simulink model "ADCS_onOrbit_TrueState"  (R2024b)
settings: Solver=ode4  StartTime=0.0  StopTime=tspan  FixedStep=1  RelTol=1e-3
undefined symbols (not defined in the file): A_list, A_m, A_w, CD, COP, dYear, eta, J_body, J_wheels, JD0, K_d, K_p, K_w, m, mag_moment, mode, mu, n_list, p, period, q1_ini, q2_ini, q3_ini, q4_ini, r_I_ini, rE, sigma_B, sigma_b, sigma_g, sigma_S, v_I_ini, wB_1, wB_2, wB_3, wE, wW_1, wW_2, wW_3
libraries: simulink_extras x12, matrix_library x3, sharedtransform x3, simulink x1
(part 2 of 2)

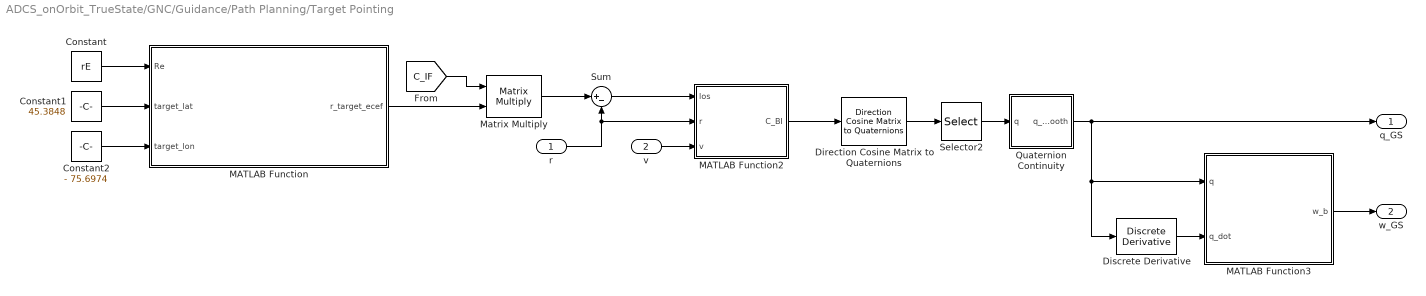
== system ADCS_onOrbit_TrueState/GNC/Guidance/Path Planning/Target Pointing ==
  r : Inport
  v : Inport  Port=2
  Constant : Constant  Value=rE
  Constant1 : Constant  Value=45.3848
  Constant2 : Constant  Value=- 75.6974
  Direction Cosine Matrix to Quaternions : sharedtransform/Direction Cosine Matrix  to Quaternions  aMode=0  action=None  tolerance=eps(2)
      settings: LibrarySourceBlock=|
      | aerolibtransform2/Direction Cosine Matrix
      | to Quaternions
  Discrete Derivative : simulink/Discrete/Discrete Derivative  gainval=1.0  ICPrevScaledInput=0.0  OutMin=[]  OutMax=[]  OutDataType=fixdt(1, 16)  OutScaling=2^-10  DoSatur=off
  MATLAB Function : MATLAB Function  TreatAsAtomicUnit=on
  MATLAB Function2 : MATLAB Function  TreatAsAtomicUnit=on
  MATLAB Function3 : MATLAB Function  TreatAsAtomicUnit=on
  Matrix Multiply : Product  Multiplication=Matrix(*)
  Quaternion Continuity : Subsystem
      mask Display: disp('Quaternion\nContinuity');
  Selector2 : Selector  InputPortWidth=4  IndexOptions=Index vector (dialog)  Indices=[2 3 4 1]  OutputSizes=1
  Sum : Sum  Inputs=|+-
  q_GS : Outport
  w_GS : Outport  Port=2
  wires:
  Constant/1 -> MATLAB Function/1(Re)
  Constant1/1 -> MATLAB Function/2(target_lat)
  Constant2/1 -> MATLAB Function/3(target_lon)
  MATLAB Function/1(r_target_ecef) -> Matrix Multiply/2
  Matrix Multiply/1 -> Sum/1
  r/1 -> MATLAB Function2/2(r), Sum/2
  Sum/1 -> MATLAB Function2/1(los)
  MATLAB Function2/1(C_BI) -> Direction Cosine Matrix to Quaternions/1
  Direction Cosine Matrix to Quaternions/1 -> Selector2/1
  Selector2/1 -> Quaternion Continuity/1(q)
  Quaternion Continuity/1(q_smooth) -> MATLAB Function3/1(q), Discrete Derivative/1, q_GS/1
  Discrete Derivative/1 -> MATLAB Function3/2(q_dot)
  MATLAB Function3/1(w_b) -> w_GS/1
  v/1 -> MATLAB Function2/3(v)
  [C_IF] -> Matrix Multiply/1

== system ADCS_onOrbit_TrueState/GNC/Navigation/TRIAD Determination/Quaternion Continuity ==
  q : Inport
  MATLAB Function2 : MATLAB Function  TreatAsAtomicUnit=on
  Unit Delay1 : UnitDelay  InitialCondition=[0 0 0 1]'  SampleTime=-1  HasFrameUpgradeWarning=on
  q_smooth : Outport
  wires:
  MATLAB Function2/1(q_smooth) -> q_smooth/1, Unit Delay1/1
  Unit Delay1/1 -> MATLAB Function2/2(q_prev)
  q/1 -> MATLAB Function2/1(q)

== system ADCS_onOrbit_TrueState/RWP/Environment/Variant Subsystem/ENV ==
  C_BI : Inport
  s : Inport  Port=2
  state : Inport  Port=3
  Drag : Subsystem
  Gravity Gradient : Subsystem
  Mag Torque : Subsystem
  Selector : Selector  InputPortWidth=6  IndexOptions=Index vector (dialog)  Indices=[1 2 3]  OutputSizes=1
  Selector1 : Selector  InputPortWidth=6  IndexOptions=Index vector (dialog)  Indices=[4 5 6]  OutputSizes=1
  Solar Radiation Pressure : Subsystem
  Sum : Sum  Inputs=++++
  B_b : Outport
  T_ext : Outport  Port=2
  a_drag : Outport  Port=3
  B_I : Outport  Port=4
  wires:
  Drag/2(a_drag) -> a_drag/1
  C_BI/1 -> Solar Radiation Pressure/1(C_BI), Drag/3(C_BI), Gravity Gradient/2(C_BI), Mag Torque/2(C_BI)
  Selector1/1 -> Drag/2(v_ECI)  "vel"
  Gravity Gradient/1(T_g) -> Sum/3
  Sum/1 -> T_ext/1  "External Torque"
  Mag Torque/1(T_mag) -> Sum/4
  Drag/1(T_atm) -> Sum/2
  Selector/1 -> Drag/1(r_ECI), Gravity Gradient/1(r_ECI), Mag Torque/1(r_ECI)  "pos"
  s/1 -> Solar Radiation Pressure/2(s)
  Mag Torque/2(B_b) -> B_b/1
  Solar Radiation Pressure/1(T_SRP) -> Sum/1
  state/1 -> Selector1/1, Selector/1
  Mag Torque/3(B_I) -> B_I/1

== system ADCS_onOrbit_TrueState/RWP/Environment/Variant Subsystem/noENV ==
  C_BI : Inport
  s : Inport  Port=2
  state : Inport  Port=3
  Constant : Constant  Value=[0; 0; 0]  VectorParams1D=off
  Constant1 : Constant  Value=[0; 0; 0]
  Mag Torque : Subsystem
  Selector : Selector  InputPortWidth=6  IndexOptions=Index vector (dialog)  Indices=[1 2 3]  OutputSizes=1
  Terminator : Terminator
  Terminator1 : Terminator
  B_b : Outport
  T_ext : Outport  Port=2
  a_drag : Outport  Port=3
  B_I : Outport  Port=4
  wires:
  Constant1/1 -> a_drag/1
  Mag Torque/1(T_mag) -> Terminator1/1
  s/1 -> Terminator/1
  C_BI/1 -> Mag Torque/2(C_BI)
  Selector/1 -> Mag Torque/1(r_ECI)  "pos"
  state/1 -> Selector/1
  Constant/1 -> T_ext/1
  Mag Torque/2(B_b) -> B_b/1
  Mag Torque/3(B_I) -> B_I/1

== system ADCS_onOrbit_TrueState/GNC/Guidance/Path Planning/Nadir Pointing/Quaternion Continuity ==
  q : Inport
  MATLAB Function2 : MATLAB Function  TreatAsAtomicUnit=on
  Unit Delay1 : UnitDelay  InitialCondition=[0 0 0 1]'  SampleTime=-1  HasFrameUpgradeWarning=on
  q_smooth : Outport
  wires:
  MATLAB Function2/1(q_smooth) -> q_smooth/1, Unit Delay1/1
  Unit Delay1/1 -> MATLAB Function2/2(q_prev)
  q/1 -> MATLAB Function2/1(q)

== system ADCS_onOrbit_TrueState/GNC/Guidance/Path Planning/Sun Pointing/Quaternion Continuity ==
  q : Inport
  MATLAB Function2 : MATLAB Function  TreatAsAtomicUnit=on
  Unit Delay1 : UnitDelay  InitialCondition=[0 0 0 1]'  SampleTime=-1  HasFrameUpgradeWarning=on
  q_smooth : Outport
  wires:
  MATLAB Function2/1(q_smooth) -> q_smooth/1, Unit Delay1/1
  Unit Delay1/1 -> MATLAB Function2/2(q_prev)
  q/1 -> MATLAB Function2/1(q)

== system ADCS_onOrbit_TrueState/GNC/Guidance/Path Planning/Target Pointing/Quaternion Continuity ==
  q : Inport
  MATLAB Function2 : MATLAB Function  TreatAsAtomicUnit=on
  Unit Delay1 : UnitDelay  InitialCondition=[0 0 0 1]'  SampleTime=-1  HasFrameUpgradeWarning=on
  q_smooth : Outport
  wires:
  MATLAB Function2/1(q_smooth) -> q_smooth/1, Unit Delay1/1
  Unit Delay1/1 -> MATLAB Function2/2(q_prev)
  q/1 -> MATLAB Function2/1(q)

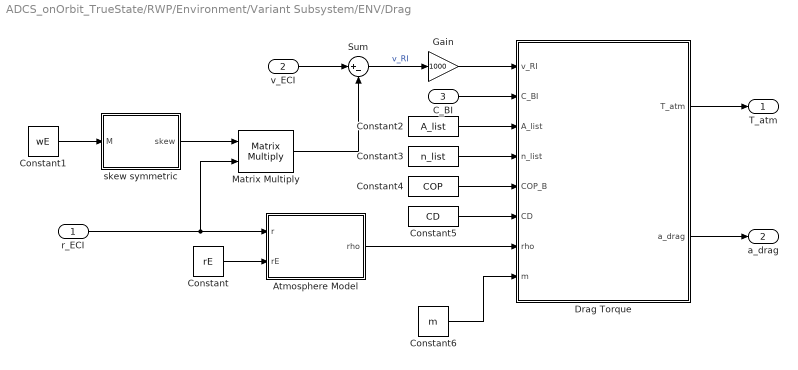
== system ADCS_onOrbit_TrueState/RWP/Environment/Variant Subsystem/ENV/Drag ==
  r_ECI : Inport
  v_ECI : Inport  Port=2
  C_BI : Inport  Port=3
  Atmosphere Model : MATLAB Function  TreatAsAtomicUnit=on
  Constant : Constant  Value=rE
  Constant1 : Constant  Value=wE
  Constant2 : Constant  Value=A_list
  Constant3 : Constant  Value=n_list
  Constant4 : Constant  Value=COP
  Constant5 : Constant  Value=CD
  Constant6 : Constant  Value=m
  Drag Torque : MATLAB Function  TreatAsAtomicUnit=on
  Gain : Gain  Gain=1000
  Matrix Multiply : Product  Multiplication=Matrix(*)
  Sum : Sum  Inputs=|+-
  skew symmetric : MATLAB Function  TreatAsAtomicUnit=on
  T_atm : Outport
  a_drag : Outport  Port=2
  wires:
  Drag Torque/2(a_drag) -> a_drag/1
  Constant6/1 -> Drag Torque/8(m)
  Atmosphere Model/1(rho) -> Drag Torque/7(rho)
  Constant5/1 -> Drag Torque/6(CD)
  Constant4/1 -> Drag Torque/5(COP_B)
  Constant3/1 -> Drag Torque/4(n_list)
  Constant2/1 -> Drag Torque/3(A_list)
  C_BI/1 -> Drag Torque/2(C_BI)
  Gain/1 -> Drag Torque/1(v_RI)
  Sum/1 -> Gain/1  "v_RI"
  v_ECI/1 -> Sum/1
  Matrix Multiply/1 -> Sum/2
  Drag Torque/1(T_atm) -> T_atm/1
  skew symmetric/1(skew) -> Matrix Multiply/1
  Constant1/1 -> skew symmetric/1(M)
  Constant/1 -> Atmosphere Model/2(rE)
  r_ECI/1 -> Atmosphere Model/1(r), Matrix Multiply/2

== system ADCS_onOrbit_TrueState/RWP/Environment/Variant Subsystem/ENV/Gravity Gradient ==
  r_ECI : Inport
  C_BI : Inport  Port=2
  Constant : Constant  Value=J_body
  Constant1 : Constant  Value=mu
  MATLAB Function3 : MATLAB Function  TreatAsAtomicUnit=on
  T_g : Outport
  wires:
  C_BI/1 -> MATLAB Function3/4(C_BI)
  Constant/1 -> MATLAB Function3/2(J)
  r_ECI/1 -> MATLAB Function3/1(r_I)
  Constant1/1 -> MATLAB Function3/3(mu)
  MATLAB Function3/1(T_g) -> T_g/1

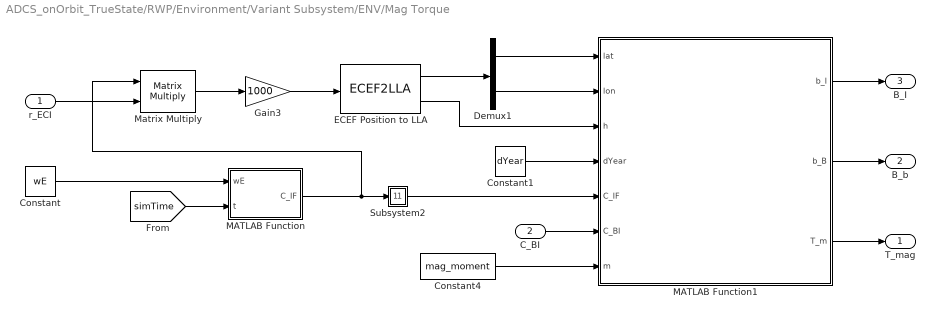
== system ADCS_onOrbit_TrueState/RWP/Environment/Variant Subsystem/ENV/Mag Torque ==
  r_ECI : Inport
  C_BI : Inport  Port=2
  Constant : Constant  Value=wE
  Constant1 : Constant  Value=dYear
  Constant4 : Constant  Value=mag_moment
  Demux1 : Demux  Outputs=2
  ECEF Position to LLA : ECEF2LLA
  Gain3 : Gain  Gain=1000
  MATLAB Function : MATLAB Function  TreatAsAtomicUnit=on
  MATLAB Function1 : MATLAB Function  TreatAsAtomicUnit=on
  Matrix Multiply : Product  Multiplication=Matrix(*)
  Subsystem2 : Subsystem
  T_mag : Outport
  B_b : Outport  Port=2
  B_I : Outport  Port=3
  wires:
  C_BI/1 -> MATLAB Function1/6(C_BI)
  Gain3/1 -> ECEF Position to LLA/1
  Matrix Multiply/1 -> Gain3/1
  r_ECI/1 -> Matrix Multiply/2
  MATLAB Function/1(C_IF) -> Matrix Multiply/1, Subsystem2/1(In1)
  Constant/1 -> MATLAB Function/1(wE)
  [simTime] -> MATLAB Function/2(t)
  ECEF Position to LLA/1 -> Demux1/1
  Demux1/1 -> MATLAB Function1/1(lat)
  Demux1/2 -> MATLAB Function1/2(lon)
  ECEF Position to LLA/2 -> MATLAB Function1/3(h)
  Constant1/1 -> MATLAB Function1/4(dYear)
  Constant4/1 -> MATLAB Function1/7(m)
  MATLAB Function1/1(b_I) -> B_I/1
  MATLAB Function1/2(b_B) -> B_b/1
  MATLAB Function1/3(T_m) -> T_mag/1
  Subsystem2/1(Out1) -> MATLAB Function1/5(C_IF)

== system ADCS_onOrbit_TrueState/RWP/Environment/Variant Subsystem/ENV/Solar Radiation Pressure ==
  C_BI : Inport
  s : Inport  Port=2
  Constant1 : Constant  Value=p
  Constant2 : Constant  Value=eta
  Constant3 : Constant  Value=A_list
  Constant4 : Constant  Value=n_list
  Constant5 : Constant  Value=COP
  MATLAB Function2 : MATLAB Function  TreatAsAtomicUnit=on
  T_SRP : Outport
  wires:
  MATLAB Function2/1(T_SRP) -> T_SRP/1
  C_BI/1 -> MATLAB Function2/7(C_BI)
  Constant5/1 -> MATLAB Function2/6(COP)
  Constant4/1 -> MATLAB Function2/5(n_list)
  Constant3/1 -> MATLAB Function2/4(A_list)
  Constant2/1 -> MATLAB Function2/3(eta)
  Constant1/1 -> MATLAB Function2/2(p)
  s/1 -> MATLAB Function2/1(r_sun)
  [inEclipse] -> MATLAB Function2/8(inEclipse)

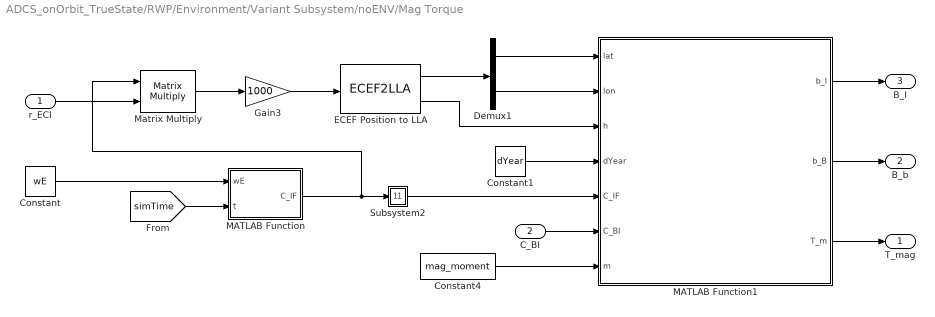
== system ADCS_onOrbit_TrueState/RWP/Environment/Variant Subsystem/noENV/Mag Torque ==
  r_ECI : Inport
  C_BI : Inport  Port=2
  Constant : Constant  Value=wE
  Constant1 : Constant  Value=dYear
  Constant4 : Constant  Value=mag_moment
  Demux1 : Demux  Outputs=2
  ECEF Position to LLA : ECEF2LLA
  Gain3 : Gain  Gain=1000
  MATLAB Function : MATLAB Function  TreatAsAtomicUnit=on
  MATLAB Function1 : MATLAB Function  TreatAsAtomicUnit=on
  Matrix Multiply : Product  Multiplication=Matrix(*)
  Subsystem2 : Subsystem
  T_mag : Outport
  B_b : Outport  Port=2
  B_I : Outport  Port=3
  wires:
  C_BI/1 -> MATLAB Function1/6(C_BI)
  Gain3/1 -> ECEF Position to LLA/1
  Matrix Multiply/1 -> Gain3/1
  r_ECI/1 -> Matrix Multiply/2
  MATLAB Function/1(C_IF) -> Matrix Multiply/1, Subsystem2/1(In1)
  Constant/1 -> MATLAB Function/1(wE)
  [simTime] -> MATLAB Function/2(t)
  ECEF Position to LLA/1 -> Demux1/1
  Demux1/1 -> MATLAB Function1/1(lat)
  Demux1/2 -> MATLAB Function1/2(lon)
  ECEF Position to LLA/2 -> MATLAB Function1/3(h)
  Constant1/1 -> MATLAB Function1/4(dYear)
  Constant4/1 -> MATLAB Function1/7(m)
  MATLAB Function1/1(b_I) -> B_I/1
  MATLAB Function1/2(b_B) -> B_b/1
  MATLAB Function1/3(T_m) -> T_mag/1
  Subsystem2/1(Out1) -> MATLAB Function1/5(C_IF)

== system ADCS_onOrbit_TrueState/RWP/Environment/Variant Subsystem/ENV/Mag Torque/Subsystem2 ==
  In1 : Inport
  Out1 : Outport
  tag scope: C_IF=global
  wires:
  In1/1 -> [C_IF], Out1/1

== system ADCS_onOrbit_TrueState/RWP/Environment/Variant Subsystem/noENV/Mag Torque/Subsystem2 ==
  In1 : Inport
  Out1 : Outport
  tag scope: C_IF=global
  wires:
  In1/1 -> [C_IF], Out1/1

== matlab function ADCS_onOrbit_TrueState/RWP/Orbit Propator/MATLAB Function1 ==
  data: t input; r_SI output; JD0 input
function r_SI = sun_vector(t, JD0)

    JD = JD0 + 1.157e-05*t;
    TUT = (JD-2451545)/36525;
    mean_long = 280.4606184 + 36000.77005361*TUT;
    mean_anom = 357.5277233 + 35999.0534*TUT;
    obliquity = 23.439291 - 0.0130042*TUT;
    lambda_e = mean_long + 1.914666471 * sind(mean_anom) + 0.019994643 * sind(2*mean_anom);
    r_sun_norm = (1.000140612 - 0.016708617 * cosd(mean_anom) + 0.019994643 * sind(2*mean_anom)) * 149597870.691; % km
    r_SI = r_sun_norm * [cosd(lambda_e); cosd(obliquity) * sind(lambda_e); sind(obliquity) * sind(lambda_e)];

end

== matlab function ADCS_onOrbit_TrueState/GNC/Guidance/Path Planning/Nadir Pointing/Quaternion Continuity/MATLAB Function2 ==
  data: q input; q_smooth output; q_prev input
function q_smooth = continuity(q, q_prev)

    if dot(q, q_prev) < 0
        q_smooth = -q;
    else
        q_smooth = q;
    end
end

== matlab function ADCS_onOrbit_TrueState/GNC/Guidance/Path Planning/Sun Pointing/Quaternion Continuity/MATLAB Function2 ==
  data: q input; q_smooth output; q_prev input
function q_smooth = continuity(q, q_prev)

    if dot(q, q_prev) < 0
        q_smooth = -q;
    else
        q_smooth = q;
    end
end

== matlab function ADCS_onOrbit_TrueState/GNC/Navigation/Subsystem/MATLAB Function2 ==
  data: q input; roll output; pitch output; yaw output; C_QI input
function [roll, pitch, yaw] = fcn(q, C_QI)

    E = q(1:3);
    n = q(4);

    C_BI = (n^2 - E'*E) * eye(3) + 2*(E*E') - 2*n*skew(E);
    C_BQ = C_BI * C_QI';
    
    roll    = atan2(C_BQ(2,3),C_BQ(3,3));
    pitch   = -asin(C_BQ(1,3));
    yaw     = atan2(C_BQ(1,2),C_BQ(1,1));

end

== matlab function ADCS_onOrbit_TrueState/GNC/Guidance/Path Planning/Target Pointing/MATLAB Function2 ==
  data: los input; C_BI output; r input; v input
function C_BI = fcn(los, r, v)

    los = los / norm(los);
    
    z_orb = los;

    y_orb = cross(v, r) / norm(cross(v,r)); % orbit normal
    y_orb = y_orb / norm(y_orb);

    x_orb = cross(y_orb, z_orb); 
    x_orb = x_orb / norm(x_orb);
    
    C_BI = [x_orb, y_orb, z_orb]';

end

== matlab function ADCS_onOrbit_TrueState/GNC/Guidance/Path Planning/Target Pointing/Quaternion Continuity/MATLAB Function2 ==
  data: q input; q_smooth output; q_prev input
function q_smooth = continuity(q, q_prev)

    if dot(q, q_prev) < 0
        q_smooth = -q;
    else
        q_smooth = q;
    end
end

== matlab function ADCS_onOrbit_TrueState/GNC/Guidance/Error/Error Quaternion ==
  data: q input; delta_q output; q_d input
function delta_q = error_quaternion(q, q_d)
% Nimish Dhawan 2025

    q_tilde = zeros(4, 4);

    q_d_conj = [-q_d(1:3); q_d(4)];

    E = q(1:3);

    E_skew = [ 0   -E(3)  E(2);
             E(3)    0   -E(1);
            -E(2)  E(1)    0  ];
    Eta = q(4);

    q_tilde = [Eta*eye(3)-E_skew, E; -E', Eta];

    delta_q = q_tilde * q_d_conj;

end

== matlab function ADCS_onOrbit_TrueState/GNC/Guidance/Error/MATLAB Function ==
  data: q_error input; theta_e output
function theta_e = pointing_error(q_error)

    q_error = q_error/norm(q_error);
    q4 = q_error(4);
    
    theta_e = rad2deg(2*acos(q4));

end

== matlab function ADCS_onOrbit_TrueState/GNC/Guidance/Path Planning/Target Pointing/MATLAB Function3 ==
  data: q input; w_b output; q_dot input
function w_b = fcn(q, q_dot)

    E = q(1:3);     % vector part of quaternion
    n = q(4);       % scalar part

    E_skew = [  0     -E(3)   E(2);
              E(3)     0    -E(1);
             -E(2)   E(1)    0  ];

    % Construct 4x3 Omega matrix
    Omega = [0.5 * (n * eye(3) + E_skew);   
             -0.5 * E'];                   

    w_b = Omega \ q_dot;   % Use backslash for stability instead of inv()

end

== matlab function ADCS_onOrbit_TrueState/GNC/Guidance/Subsystem3/MATLAB Function1 ==
  data: q input; roll output; pitch output; yaw output
function [roll, pitch, yaw] = fcn(q)

    E = q(1:3);
    n = q(4);

    C_BI = (n^2 - E'*E) * eye(3) + 2*(E*E') - 2*n*skew(E);

    roll    = atan2(C_BI(2,3),C_BI(3,3));
    pitch   = -asin(C_BI(1,3));
    yaw     = atan2(C_BI(1,2),C_BI(1,1)); 


end

== matlab function ADCS_onOrbit_TrueState/RWP/Orbit Propator/MATLAB Function2 ==
  data: r_S input; s output
function s = fcn(r_S)

s = r_S/norm(r_S);

== matlab function ADCS_onOrbit_TrueState/RWP/Environment/Variant Subsystem/ENV/Mag Torque/MATLAB Function1 ==
  data: lat input; b_I output; lon input; h input; dYear input; C_IF input; C_BI input; m input; b_B output; T_m output
function [b_I, b_B, T_m] = fcn(lat, lon, h, dYear, C_IF, C_BI, m)

    coder.extrinsic('wrldmagm');
    
    % dYear = 2025.0;
    b = zeros(3,1);
    lat_geo = lat;

    m_skew = [0     m(3) -m(2)
             -m(3)  0     m(1)
              m(2) -m(1)  0  ];
    
    % World Magnetic Model
    % [b, H, DEC, DIP, F] = wrldmagm(h, lat, lon, dYear,'Custom','WMM2025.COF');
    [b, H, DEC, DIP, F] = wrldmagm(h, lat, lon, dYear, 2020);

    % Conversion to go from NED to ECEF
    sLat = sind(lat_geo);
    cLat = cosd(lat_geo);

    sLon = sind(lon);
    cLon = cosd(lon);
 
    C_FN = [-sLat*cLon -sLat*sLon cLat; -sLon cLon 0; -cLat*cLon -cLat*sLon -sLat]';
    b_ECEF = C_FN * b;

    % Going from ECEF to ECI
    b_I = C_IF * b_ECEF;

    % Conversion to Body Frame
    b_B = C_BI * b_I;

    % Magnetic Torque
    T_m = m_skew * b_B * 1e-09;

end

== matlab function ADCS_onOrbit_TrueState/RWP/Nonlinear Spacecraft/Spacecraft Dynamics/MATLAB Function1 ==
  data: h_tot input; T_b input; h_tot_dot output; J input; A_w input; h_w input; w_b output
function [h_tot_dot, w_b] = dynamics(h_tot, T_b, J, A_w, h_w)

% Nimish Dhawan 2025

% T_b : net body torque (ext + MTQ - wheel torque on body)      [3x1]
% J     : body inertia                                          [3x3]
% A_w   : wheel axis matrix (columns = wheel axes, body frame)  [3x3]
% h_w   : wheel angular momentum                                [3x1]
% h_tot : current total angular momentum of SC (state)          [3x1]

% ---- omega from momentum ----
w_b = J \ (h_tot - A_w * h_w);       

% ---- h_tot dynamics ----
h_tot_dot = T_b - skew(w_b) * h_tot;

end

== matlab function ADCS_onOrbit_TrueState/RWP/Nonlinear Spacecraft/Spacecraft Kinematics/MATLAB Function1 ==
  data: q input; q_dot output; w input
function q_dot = kinematics(q, w)

% Nimish Dhawan 2025
% Input: 
% q = quaternion (4x1) [scalar last]
% w = angular velocity of s/c (3x1) [SBF]

E   = q(1:3);
Eta = q(4);

E_dot   = 0.5 * (Eta*eye(3) + skew(E)) * w;
Eta_dot = -0.5 * (E' * w); 

q_dot = [E_dot; Eta_dot];

end

== matlab function ADCS_onOrbit_TrueState/RWP/Nonlinear Spacecraft/Spacecraft Kinematics/Quaternion Normalize1 ==
  data: q input; q_norm output
function q_norm = q_normalize(q)

q_norm = q/norm(q);

== matlab function ADCS_onOrbit_TrueState/RWP/Orbit Propator/Two Body/MATLAB Function1 ==
  data: r_I input; a_I output; mu input
function a_I = fcn(r_I, mu)

a_I = r_I .* (-mu / (norm(r_I)^3));

end

== matlab function ADCS_onOrbit_TrueState/RWP/Orbit Propator/Two Body/MATLAB Function3 ==
  data: r input; a_j2 output; mu input; rE input
function a_j2 = J2_perturbation(r, mu, rE)

    J2 = 1.08263e-3;

    x = r(1); y = r(2); z = r(3);
    r_norm = norm(r);

    factor = -(3/2) * J2 * mu * rE^2 / r_norm^5;
    zx2_r2 = 5*z^2 / r_norm^2;

    a_j2 = factor * [
        x * (1 - zx2_r2);
        y * (1 - zx2_r2);
        z * (3 - zx2_r2)
    ];
    
end

== matlab function ADCS_onOrbit_TrueState/RWP/Orbit Propator/MATLAB Function ==
  data: q input; C_BI output
function C_BI = QUAT2DCM(q)

% Nimish Dhawan
% 2025

%%%%%%%%%%%%%%%%%%%%%%%%%%%%%%%%%%%%%%%%%%%%%%%%%%%%%%%%%%%%%%%%%%%%%%%%%
% Input(s)
%%%%%%%%%%%%%%%%%%%%%%%%%%%%%%%%%%%%%%%%%%%%%%%%%%%%%%%%%%%%%%%%%%%%%%%%%
% q (4x1): Quaternion

%%%%%%%%%%%%%%%%%%%%%%%%%%%%%%%%%%%%%%%%%%%%%%%%%%%%%%%%%%%%%%%%%%%%%%%%%
% Output(s)
%%%%%%%%%%%%%%%%%%%%%%%%%%%%%%%%%%%%%%%%%%%%%%%%%%%%%%%%%%%%%%%%%%%%%%%%%
% C_BI (3x3): Rotation matrix to go from ECI to Body Fixed Frame

E = q(1:3);
Eta = q(4);

C_BI = (Eta^2-E'*E)*eye(3) + 2*(E*E') - 2*Eta*skew(E);

== matlab function ADCS_onOrbit_TrueState/OBC/RES/MATLAB Function ==
  data: u input; y output
function y = magnitude(u)

y = norm(u);

== matlab function ADCS_onOrbit_TrueState/ACT/Wheels + Magnetorquers/Wheel 1/MATLAB Function1 ==
  data: h_wi output; w_wi output; J_w input; h_w input; wB input; A_w input
function [h_wi, w_wi] = fcn(J_w, h_w, wB, A_w)

% Nimish Dhawan 2025

i       = 1;      % Wheel No.

J_inv   = 1 / J_w;
Aw_i    = [A_w(:,i)];
h_wi    = h_w ;

w_wi = J_inv * h_wi * Aw_i - Aw_i' * wB;

end

== matlab function ADCS_onOrbit_TrueState/ACT/Wheels + Magnetorquers/Wheel 2/MATLAB Function1 ==
  data: h_wi output; w_wi output; J_w input; h_w input; wB input; A_w input
function [h_wi, w_wi] = fcn(J_w, h_w, wB, A_w)

% Nimish Dhawan 2025

i       = 2;      % Wheel No.

J_inv   = 1 / J_w;
Aw_i    = [A_w(:,i)];
h_wi    = h_w ;

w_wi = J_inv * h_wi * Aw_i - Aw_i' * wB;

end

== matlab function ADCS_onOrbit_TrueState/RWP/Environment/MATLAB Function ==
  data: u input; y output
function y = magnitude(u)

y = norm(u);

== matlab function ADCS_onOrbit_TrueState/ACT/Wheels + Magnetorquers/Wheel 3/MATLAB Function1 ==
  data: h_wi output; w_wi output; J_w input; h_w input; wB input; A_w input
function [h_wi, w_wi] = fcn(J_w, h_w, wB, A_w)

% Nimish Dhawan 2025

i       = 3;      % Wheel No.

J_inv   = 1 / J_w;
Aw_i    = [A_w(:,i)];
h_wi    = h_w ;

w_wi = J_inv * h_wi * Aw_i - Aw_i' * wB;

end

== matlab function ADCS_onOrbit_TrueState/RWP/Environment/Variant Subsystem/ENV/Gravity Gradient/MATLAB Function3 ==
  data: r_I input; J input; mu input; C_BI input; T_g output
function T_g = fcn(r_I, J, mu, C_BI)

r_B = C_BI * r_I;
r = norm(r_I);

T_g = (3*mu/r^5) * skew(r_B) * J * r_B;

== matlab function ADCS_onOrbit_TrueState/ACT/Wheels + Magnetorquers/Reaction Wheel Power/MATLAB Function3 ==
  data: Tc input; Prw output; h_W input; Ptotal output; P_pre input
function [Prw, Ptotal]= fcn(Tc, h_W, P_pre)

% Nimish Dhawan
% Reaction wheel power consumption as given in "Comarison of Control Moment
% Gyros and Reaction Wheels for Small Earth-Observing Satellites


% Eq. 3
alpha = 0.47;     % empirical exponent
k2    = 4.51;     % empirical coeff

Prw = 1000.*abs(Tc) + k2.*(abs(h_W).^(alpha));   % per-wheel power [W]
Ptotal = (P_pre + Prw); 

end

== matlab function ADCS_onOrbit_TrueState/GNC/Controller/Torque Saturation/Slew Limit ==
  data: Tcmd input; Tlim output; ts input; Tdot_max input; T_prev input
function Tlim = fcn(Tcmd, ts, Tdot_max, T_prev)

    Tdelta = Tcmd - T_prev;
    deltaMax = Tdot_max * ts;
    Tdelta_sat = zeros(3,1);

    for i = 1:3    
        if abs(Tdelta(i)) > deltaMax
            Tdelta_sat(i) = sign(Tdelta(i)) * deltaMax;
        else
            Tdelta_sat(i) = Tdelta(i); 
        end
    end

    Tlim = T_prev + Tdelta_sat;

end

== matlab function ADCS_onOrbit_TrueState/ACT/Wheels + Magnetorquers/MATLAB Function ==
  data: T_c input; T_cmd output; wheelsEnabled input
function T_cmd = fcn(T_c, wheelsEnabled)

if wheelsEnabled == 1
    T_cmd = T_c;
else
    T_cmd = [0; 0; 0];
end

end

== matlab function ADCS_onOrbit_TrueState/RWP/Environment/Variant Subsystem/ENV/Drag/Atmosphere Model ==
  data: rho output; r input; rE input
function rho = atmosphere(r, rE)

    z = norm(r)-rE;        % Altitude (km) 
    
    if 400 <= z && z < 450
        rho0 = 3.275e-12;
        h0   = 400;
        H    = 58.515;
    elseif 450 <= z && z < 500
        rho0 = 1.585e-12;   % kg/m³
        h0   = 450;   % km
        H    = 60.828;  % km
    elseif 500 <= z && z < 600
        rho0 = 6.967e-13;   % kg/m³
        h0   = 500;   % km
        H    = 63.822;  % km
    elseif 600 <= z && z < 700
        rho0 = 1.454e-13;
        h0   = 600;
        H    = 71.835;
    elseif 700 <= z && z < 800
        rho0 = 3.614e-14;
        h0   = 700;
        H    = 88.667;
    else
        rho0 = 1.170e-14;
        h0   = 800;
        H    = 124.64;
    end

    rho = rho0 * exp(-(z-h0)/H);    % in kg/m³

end

== matlab function ADCS_onOrbit_TrueState/RWP/Environment/Variant Subsystem/ENV/Drag/Drag Torque ==
  data: v_RI input; C_BI input; A_list input; n_list input; COP_B input; CD input; T_atm output; rho input; a_drag output; m input
function [T_atm, a_drag] = drag_torque(v_RI, C_BI, A_list, n_list, COP_B, CD, rho, m)

    v_RI_hat = v_RI / norm(v_RI);     
    v_RI_mag = norm(v_RI);            
    T_atm = [0; 0; 0];
    F_drag = [0; 0; 0];
    a_drag = [0; 0; 0];

    for k = 1:length(A_list)
        n_k = n_list(k, :).';         
        A_k = A_list(k);              

        cos_alpha_k = dot(n_k, C_BI * v_RI_hat);

        if cos_alpha_k > 0
            F_k = - 0.5 * rho * CD * A_k * v_RI_mag^2 * cos_alpha_k * v_RI_hat;
        else 
            F_k = [0; 0; 0];
        end
        F_drag = F_drag + F_k;
        a_drag = F_drag/m;

        F_k_B = C_BI * F_k;
        COP_B_k = COP_B(k, :).';
        T_k = cross(COP_B_k, F_k_B);
        T_atm = T_atm + T_k;
    end

end

== matlab function ADCS_onOrbit_TrueState/RWP/Environment/Variant Subsystem/ENV/Drag/skew symmetric ==
  data: M input; skew output
function skew = skew_matrix(M)

    skew = [0 M(3) -M(2)
            -M(3) 0 M(1)
            M(2) -M(1) 0];

end

== matlab function ADCS_onOrbit_TrueState/GNC/Navigation/MEKF/MATLAB Function ==
  data: q_pre input; w_meas input; b_pre input; dt input; s_I input; b_I input; s_B input; b_B input; R input; sigma_g input; sigma_b input; q_plus output; b_plus output; P_pre input; P_plus output
function [q_plus, b_plus, P_plus] = fcn(q_pre, w_meas, b_pre, dt, s_I, ...
                                b_I, s_B, b_B, R, sigma_g, sigma_b, P_pre)
% Nimish Dhawan 2025

%%%%%%%%%%%%%%%%%%%%%%%%%%%%%%%%%%%%%%%%%%%%%%%%%%%%%%%%%%%%%%%%%%%%%%%%%
% Input(s)
%%%%%%%%%%%%%%%%%%%%%%%%%%%%%%%%%%%%%%%%%%%%%%%%%%%%%%%%%%%%%%%%%%%%%%%%%


%%%%%%%%%%%%%%%%%%%%%%%%%%%%%%%%%%%%%%%%%%%%%%%%%%%%%%%%%%%%%%%%%%%%%%%%%
% Output(s)
%%%%%%%%%%%%%%%%%%%%%%%%%%%%%%%%%%%%%%%%%%%%%%%%%%%%%%%%%%%%%%%%%%%%%%%%%

tilde  = @(E, Eta) [Eta*eye(3)-skew(E), E; -E', Eta];
qBox   = @(E, Eta) [Eta*eye(3)+skew(E), E; -E', Eta];
qDot   = @(q, w) 0.5 * qBox(q(1:3), q(4)) * [w; 0];
quat2C = @(E, Eta) (Eta^2-E'*E)*eye(3) + 2*(E*E') - 2*Eta*skew(E);

s_I = s_I/norm(s_I);
s_B = s_B/norm(s_B);
b_I = b_I/norm(b_I);
b_B = b_B/norm(b_B);

% ========================================================================
% Propagation
w_hat = w_meas - b_pre;
db    = zeros(3,1);          % Mean is zero, covariance accounted for in Q

% phi = norm(w_hat)*dt;
% phi = (w_hat)*dt/100;
phi = zeros(3,1);


dq = [0.5*phi; 1];

% q_minus is quat multipication of q_predicted using q_pre
k1 = qDot(q_pre          , w_hat);
k2 = qDot(q_pre+0.5*k1*dt, w_hat);
k3 = qDot(q_pre+0.5*k2*dt, w_hat);
k4 = qDot(q_pre+k3*dt    , w_hat);

q_pred = q_pre + (dt/6)*(k1+2*k2+2*k3+k4); 
q_pred = q_pred/norm(q_pred);

% Priori Estimates
q_minus = tilde(dq(1:3), dq(4)) * q_pred;
q_minus = q_minus/norm(q_minus);
b_minus = b_pre + db;

Phi11 = eye(3) - (1/norm(w_hat))*skew(w_hat)*sin(phi) + ...
        (1/norm(w_hat))^2*skew(w_hat)^2*(1-cos(phi));
Phi12 = -eye(3)*dt - (1/norm(w_hat))^2*skew(w_hat)^3*(phi-sin(phi)) + ...
        (1/norm(w_hat))*skew(w_hat)^2*(1-cos(phi));
Phi   = [Phi11, Phi12; zeros(3,3), eye(3,3)];

Q11 = (sigma_g^2*dt + sigma_b^2*dt^3/3) * eye(3);
Q12 = -(sigma_b^2*dt^2/2) * eye(3);
Q22 = sigma_g^2*dt * eye(3);
Q   = [Q11, Q12; Q12, Q22];

% Priori Covariance
P_minus = Phi*P_pre*Phi' + Q;

% ========================================================================
% Correction
C_BI = quat2C(q_minus(1:3), q_minus(4));

% Predicted Measurement
h = [C_BI*s_I;
     C_BI*b_I];

% Measurement Jacobian
H = [skew(C_BI*s_I), zeros(3,3);
     skew(C_BI*b_I), zeros(3,3)];

% Measurement
z = [s_B;
     b_B];

% Residual
r = z - h;

% Kalman Gain
S = H*P_minus*H' + R;
K = P_minus * H' * inv(S);

dx_plus     = K*r;
dth_plus    = dx_plus(1:3);
dq_plus     = [0.5*dth_plus; 1];
dq_plus     = dq_plus / norm(dq_plus);
db_plus     = dx_plus(4:6);

P_plus = P_minus * (eye(6) - K*H);
% P_plus = (eye(6) - K*H) * P_minus * (eye(6) - K*H)' + K*R*K';

% Reset
q_plus = tilde(dq_plus(1:3), dq_plus(4)) * q_minus;
q_plus = q_plus / norm(q_plus);
b_plus = b_minus + db_plus;


end

== matlab function ADCS_onOrbit_TrueState/RWP/Orbit Propator/Eclipse Detection/MATLAB Function3 ==
  data: R_s input; eclipse_entry output; r_sat input; r_E input; was_in_eclipse input; eclipse_exit output; is_in_eclipse output
function [eclipse_entry, eclipse_exit, is_in_eclipse] = fcn(R_s, r_sat, r_E, was_in_eclipse)

    % Convert input to numeric (if it came in as logical)
    if was_in_eclipse
        was = 1;
    else
        was = 0;
    end

    % Normalize sun vector
    s_hat = R_s / norm(R_s);

    % Projection of satellite position onto sun vector
    proj = dot(r_sat, s_hat);
    closest_point = proj * s_hat;

    % Perpendicular distance from Earth center to Sun-sat line
    d = norm(r_sat - closest_point);

    % Check if satellite is in eclipse
    if (d < r_E) && (proj < 0)
        is_in_eclipse = 1;
    else
        is_in_eclipse = 0;
    end

    % Detect eclipse entry
    if (was == 0) && (is_in_eclipse == 1)
        eclipse_entry = 1;
    else
        eclipse_entry = 0;
    end

    % Detect eclipse exit
    if (was == 1) && (is_in_eclipse == 0)
        eclipse_exit = 1;
    else
        eclipse_exit = 0;
    end

end

== matlab function ADCS_onOrbit_TrueState/SENS/Gyroscope/MATLAB Function1 ==
  data: w_sc input; w_meas output; bias input; noise input
function w_meas = fcn(w_sc, bias, noise)

rand_w = noise .* ones(3,1);
bias   = bias .* ones(3,1);

w_meas = w_sc + bias + rand_w;

== matlab function ADCS_onOrbit_TrueState/GNC/Guidance/Path Planning/Nadir Pointing/ECI to SB ==
  data: r input; C_BI output; v input
function C_BI = fcn(r, v)

    % Converts vectors in ECI to Spacecraft Body Frame

    r = r(:); v = v(:);
    
    z_orb = - r / norm(r);                  % nadir
    y_orb = cross(v, r) / norm(cross(v,r)); % orbit normal
    y_orb = y_orb / norm(y_orb);

    x_orb = cross(y_orb, z_orb); 
    x_orb = x_orb / norm(x_orb);

    C_BI = [x_orb, y_orb, z_orb]';
end

== matlab function ADCS_onOrbit_TrueState/RWP/Nonlinear Spacecraft/Subsystem/MATLAB Function2 ==
  data: q input; roll output; pitch output; yaw output; C_QI input
function [roll, pitch, yaw] = fcn(q, C_QI)

    E = q(1:3);
    n = q(4);

    C_BI = (n^2 - E'*E) * eye(3) + 2*(E*E') - 2*n*skew(E);
    C_BQ = C_BI * C_QI';
    
    roll    = atan2(C_BQ(2,3),C_BQ(3,3));
    pitch   = -asin(C_BQ(1,3));
    yaw     = atan2(C_BQ(1,2),C_BQ(1,1));

end

== matlab function ADCS_onOrbit_TrueState/GNC/Navigation/Subsystem1/MATLAB Function2 ==
  data: q input; roll output; pitch output; yaw output; C_QI input
function [roll, pitch, yaw] = fcn(q, C_QI)

    E = q(1:3);
    n = q(4);

    C_BI = (n^2 - E'*E) * eye(3) + 2*(E*E') - 2*n*skew(E);
    C_BQ = C_BI * C_QI';
    
    roll    = atan2(C_BQ(2,3),C_BQ(3,3));
    pitch   = -asin(C_BQ(1,3));
    yaw     = atan2(C_BQ(1,2),C_BQ(1,1));

end

== matlab function ADCS_onOrbit_TrueState/GNC/Guidance/Path Planning/Sequence Logic ==
  data: q_GC input; w_GC input; q_nadir input; q output; w_nadir input; q_sun input; w_sun input; t input; opMode input; in_eclipse input; w output; eclipse_exit input; mode output; t_eclipse_exit_prev input; t_eclipse_exit_out output
function [q, w, mode, t_eclipse_exit_out] = fcn(q_GC, w_GC, q_nadir, w_nadir, q_sun, w_sun, t, opMode, in_eclipse, eclipse_exit, t_eclipse_exit_prev)

    option = opMode;
    q = zeros(4,1);
    w = zeros(3,1);
    mode = 0;

    % Store new eclipse exit time if just exited
    if eclipse_exit == 1
        t_eclipse_exit_out = t;
    else
        t_eclipse_exit_out = t_eclipse_exit_prev;
    end

    % Manual override modes
    % For mission mode, detumble mode, desaturation mode and safemode
    if option ~= 1 && option ~= 2 && option ~= 3
        q = q_nadir;
        w = w_nadir;
        mode = 0;

    % For comms mode
    elseif option == 3
        q = q_GC;
        w = w_GC;
       
    % Idle mode
    elseif option == 1
        q = q_sun;
        w = w_sun;
        mode = 1;

    % Auto switch mode
    elseif option == 2
        if in_eclipse == 1
            q = q_sun;
            w = w_sun;
            mode = 1;
        else
            if t <= (t_eclipse_exit_out + 30*60)
                q = q_sun;
                w = w_sun;
                mode = 1;
            else
                q = q_nadir;
                w = w_nadir;
                mode = 0;
            end
        end
    end

end

== matlab function ADCS_onOrbit_TrueState/RWP/Environment/Variant Subsystem/ENV/Mag Torque/MATLAB Function ==
  data: wE input; C_IF output; t input
function C_IF = fcn(wE, t)

    theta = wE(3) * t;

    C_IF = [cos(theta) sin(theta) 0; -sin(theta) cos(theta) 0; 0 0 1]';

end

== matlab function ADCS_onOrbit_TrueState/GNC/Guidance/Path Planning/Sun Pointing/MATLAB Function ==
  data: q output; DCM input
function q = dcm2quat(DCM)
    A = DCM;
    q = zeros(4,1); % [q1; q2; q3; q4] — vector-first

    tr = trace(A);

    if tr > 0
        S = sqrt(tr + 1.0) * 2; % S = 4*q4
        q(4) = 0.25 * S;
        q(1) = (A(3,2) - A(2,3)) / S;
        q(2) = (A(1,3) - A(3,1)) / S;
        q(3) = (A(2,1) - A(1,2)) / S;
    elseif (A(1,1) > A(2,2)) && (A(1,1) > A(3,3))
        S = sqrt(1.0 + A(1,1) - A(2,2) - A(3,3)) * 2; % S = 4*q1
        q(1) = 0.25 * S;
        q(2) = (A(1,2) + A(2,1)) / S;
        q(3) = (A(1,3) + A(3,1)) / S;
        q(4) = (A(3,2) - A(2,3)) / S;
    elseif (A(2,2) > A(3,3))
        S = sqrt(1.0 + A(2,2) - A(1,1) - A(3,3)) * 2; % S = 4*q2
        q(1) = (A(1,2) + A(2,1)) / S;
        q(2) = 0.25 * S;
        q(3) = (A(2,3) + A(3,2)) / S;
        q(4) = (A(1,3) - A(3,1)) / S;
    else
        S = sqrt(1.0 + A(3,3) - A(1,1) - A(2,2)) * 2; % S = 4*q3
        q(1) = (A(1,3) + A(3,1)) / S;
        q(2) = (A(2,3) + A(3,2)) / S;
        q(3) = 0.25 * S;
        q(4) = (A(2,1) - A(1,2)) / S;
    end

    q = q / norm(q); % normalize
end

== matlab function ADCS_onOrbit_TrueState/RWP/Environment/Variant Subsystem/ENV/Solar Radiation Pressure/MATLAB Function2 ==
  data: r_sun input; T_SRP output; p input; eta input; A_list input; n_list input; COP input; C_BI input; inEclipse input
function T_SRP = fcn(r_sun, p, eta, A_list, n_list, COP, C_BI, inEclipse)

    T_SRP = [0; 0; 0];
    r_sun = r_sun(:);  

    for k = 1:length(A_list)
        n_k = n_list(k, :)';          % column vector (3x1)
        A_k = A_list(k);              % scalar area

        cos_alpha_k = dot(n_k, C_BI * r_sun);  

        if cos_alpha_k > 0 && inEclipse == 0
            F_srp_k = -p * A_k * eta * cos_alpha_k * r_sun;  
        else
            F_srp_k = [0; 0; 0];
        end

        F_srp_k_B = C_BI * F_srp_k;
        COP_k = COP(k, :)';
        T_SRP_k = cross(COP_k, F_srp_k_B);

        T_SRP = T_SRP + T_SRP_k;
    end

end

== matlab function ADCS_onOrbit_TrueState/GNC/Guidance/Path Planning/Sun Pointing/MATLAB Function2 ==
  data: s_i input; C_BI output
function C_BI = fcn(s_i)

    % Ecliptic notth pole
    epsilon = deg2rad(23.44);  % Obliquity of the ecliptic
    n_ecl = [0; -sin(epsilon); cos(epsilon)];

    x_b = s_i / norm(s_i);
    z_b = n_ecl - dot(n_ecl, x_b) * x_b; % Gram-Schmidt orthogonalization
    z_b = z_b / norm(z_b); 
    if dot(z_b, n_ecl) < 0
        z_b = -z_b; 
    end
    y_b = cross(z_b, x_b);
    
    C1 = [x_b y_b z_b];   

    theta = deg2rad(45);

    Rz = [cos(theta), -sin(theta), 0;
          sin(theta),  cos(theta), 0;
          0,           0,          1];
    
    C_BI = C1 * Rz';

end

== matlab function ADCS_onOrbit_TrueState/GNC/Navigation/TRIAD Determination/Quaternion Continuity/MATLAB Function2 ==
  data: q input; q_smooth output; q_prev input
function q_smooth = continuity(q, q_prev)

    if dot(q, q_prev) < 0
        q_smooth = -q;
    else
        q_smooth = q;
    end
end

== matlab function ADCS_onOrbit_TrueState/GNC/Navigation/TRIAD Determination/MATLAB Function1 ==
  data: s_I input; C_BI output; m_I input; s_b input; m_b input
function C_BI = fcn(s_I, m_I, s_b, m_b)

% Normalizing vectors
sI = s_I/norm(s_I);
sB = s_b/norm(s_b);
mI = m_I/norm(m_I);
mB = m_b/norm(m_b);

% Determining M_I 
r1 = sI;
r2 = cross(sI,mI)/norm(cross(sI,mI));
r3 = cross(r1, r2);
MI = [r1, r2, r3];

% Determining M_B
s1 = sB;
s2 = cross(sB,mB)/norm(cross(sB,mB));
s3 = cross(s1, s2);

MB = [s1, s2, s3]; 

C_BI = MB * transpose(MI);

end

== matlab function ADCS_onOrbit_TrueState/SENS/Gyroscope/MATLAB Function ==
  data: biasDot output; noise input
function biasDot = fcn(noise)

bias_noise = noise.*[1;1;1];

biasDot = bias_noise;

== matlab function ADCS_onOrbit_TrueState/GNC/Controller/MATLAB Function ==
  data: opMode input; t input; T_w output; period input; B_meas input; w input; J_body input; K_p input; K_d input; K_w input; q_error input; w_error input; h_w input; M output
function [T_w, M] = fcn(opMode ,t, period, B_meas, w, J_body, K_p, K_d, K_w, q_error, w_error, h_w)

T_w = [0; 0; 0];
M = [0; 0; 0];

w_skew = skew(w);

% Modified PD control
if opMode ~= 4 && opMode ~= 5 && opMode ~= 6 && opMode ~= 7 && opMode ~= 8

    % Gain Scheduling
    theta_e = 2*atan2(norm(q_error(1:3)), q_error(4));
    wr = norm(w_error);

    Kd0 = diag(K_d*ones(3,1));
    Kp0 = diag(K_p*ones(3,1));

    % Kd0 = diag([0.01, 0.025, 0.01]);
    % Kp0 = diag([0.000125/2, 0.000125, 0.000125/2])./2;

    e1 = deg2rad(1.0);
    e2 = deg2rad(3.0);
    w1 = deg2rad(0.05);
    w2 = deg2rad(0.1);

    % alpha_p = (theta_e < e1)*0.6 + (theta_e >= e1 && theta_e < e2)*5.0 + (theta_e >= e2)*1.6;
    % alpha_d = (wr < w1)*0.9 + (wr >= w1 && wr < w2)*1.2 + (wr >= w2)*1.6;

    alpha_p = (theta_e < e1)*0.6 + (theta_e >= e1 && theta_e < e2 && opMode == 0)*5.0 + ...
                (theta_e >= e1 && theta_e < e2 && opMode == 1)*0.2 + (theta_e >= e2)*1;
    alpha_d = (wr < w1)*0.9 + (wr >= w1 && wr < w2)*1.2 + (wr >= w2)*2;

    if wr >= w2
        alpha_p = 0.7*alpha_p;
        alpha_d = 1.3*alpha_d;
    end

    alpha_p = min(max(alpha_p,0.0),2.5);
    alpha_d = min(max(alpha_d,0.5),3.0);

    K_p = alpha_p*Kp0;
    K_d = alpha_d*Kd0;
        
    % K_d = diag([0.01, 0.025, 0.01]);
    % K_p = diag([0.000125/2, 0.000125, 0.000125/2])./2;

    % Control algorithm
    T_w = w_skew * J_body * w - K_p * eye(3) * q_error(1:3) - K_d * eye(3) * w_error;

% B-dot 
elseif opMode == 8
    M = -K_w * cross(B_meas, w);

% No control - Safe mode and LEOP
elseif opMode == 6 || opMode == 7
    T_w = [0; 0; 0];
    M = [0; 0; 0];

% Desaturation (incomplete)
elseif opMode == 5
    % Trigger for dumping
    if t < (12*period) && t > (10*period) % Create a proper autonomous trigger for dumping
        k_desat = -0.0005;
    else
        k_desat = 0;
    end

    % Controller gains
    K_p = 5e-4;
    K_d = 5e-05;
    
    % Desired wheel momentum [h_w1; h_w2; h_w3]
    h_wn = [0; 0; 0];
    B2 = norm(B_meas)^2;

    % Control algorithm
    T_ctrl = w_skew * J_body * w - K_p * eye(3) * q_error(1:3) - K_d * eye(3) * w_error;
    M_dump = (k_desat/B2) * (cross(B_meas, (h_w - h_wn))); 
    % T_dump = cross(M_dump, B_meas);

    T_w = T_ctrl;
    M = M_dump;
    % T_mag = T_dump;
    % 
    % M = (1/B2) * cross(B_meas, T_mag);

% Simple Bdot Detumble (works)
elseif opMode == 4
    wr = norm(w_error);
    if t > 200 % t < (1*period) && 
        Kw0 = K_w;
        alpha = (wr > deg2rad(1)) * 5 + (wr <= deg2rad(1)) * 10;
        Kw = alpha*Kw0;
        M = - Kw * cross(B_meas, w);
        T_w = [0; 0; 0];
    elseif wr < deg2rad(0.5) && norm(slewrate(w_error)) < 1        % t > 1 * period && abs(norm(w)) < 0.05
        T_w = w_skew * J_body * w - K_p * eye(3) * q_error(1:3) - K_d * eye(3) * w_error;
        M = [0; 0; 0]; 
    else
        T_w = [0; 0; 0];
        M = [0; 0; 0]; 
    end

end

end

== matlab function ADCS_onOrbit_TrueState/RWP/Environment/Variant Subsystem/noENV/Mag Torque/MATLAB Function ==
  data: wE input; C_IF output; t input
function C_IF = fcn(wE, t)

    theta = wE(3) * t;

    C_IF = [cos(theta) sin(theta) 0; -sin(theta) cos(theta) 0; 0 0 1]';

end

== matlab function ADCS_onOrbit_TrueState/ACT/Wheels + Magnetorquers/Magnetorquer 1/skew symmetric ==
  data: M input; skew output
function skew = skew_matrix(M)

    skew = [0 M(3) -M(2)
            -M(3) 0 M(1)
            M(2) -M(1) 0];

end

== matlab function ADCS_onOrbit_TrueState/ACT/Wheels + Magnetorquers/Magnetorquer 2/skew symmetric ==
  data: M input; skew output
function skew = skew_matrix(M)

    skew = [0 M(3) -M(2)
            -M(3) 0 M(1)
            M(2) -M(1) 0];

end

== matlab function ADCS_onOrbit_TrueState/ACT/Wheels + Magnetorquers/Magnetorquer 3/skew symmetric ==
  data: M input; skew output
function skew = skew_matrix(M)

    skew = [0 M(3) -M(2)
            -M(3) 0 M(1)
            M(2) -M(1) 0];

end

== matlab function ADCS_onOrbit_TrueState/ACT/Wheels + Magnetorquers/MATLAB Function1 ==
  data: M_c input; M_cmd output; rodsEnable input
function M_cmd = fcn(M_c, rodsEnable)

if rodsEnable == 1
    M_cmd = M_c;
else
    M_cmd = [0; 0; 0];
end

end

== matlab function ADCS_onOrbit_TrueState/RWP/Environment/Variant Subsystem/noENV/Mag Torque/MATLAB Function1 ==
  data: lat input; b_I output; lon input; h input; dYear input; C_IF input; C_BI input; m input; b_B output; T_m output
function [b_I, b_B, T_m] = fcn(lat, lon, h, dYear, C_IF, C_BI, m)

    coder.extrinsic('wrldmagm');
    
    % dYear = 2025.0;
    b = zeros(3,1);
    lat_geo = lat;

    m_skew = [0     m(3) -m(2)
             -m(3)  0     m(1)
              m(2) -m(1)  0  ];
    
    % World Magnetic Model
    [b, H, DEC, DIP, F] = wrldmagm(h, lat, lon, dYear,'2020');
    
    % Conversion to go from NED to ECEF
    sLat = sind(lat_geo);
    cLat = sind(lat_geo);

    sLon = sind(lon);
    cLon = cosd(lon);
 
    C_FN = [-sLat*cLon -sLat*sLon cLat; -sLon cLon 0; -cLat*cLon -cLat*sLon -sLat]';
    b_ECEF = C_FN * b;

    % Going from ECEF to ECI
    b_I = C_IF * b_ECEF;

    % Conversion to Body Frame
    b_B = C_BI * b_I;

    % Magnetic Torque
    T_m = m_skew * b_B * 1e-09;

end

== matlab function ADCS_onOrbit_TrueState/GNC/Guidance/Path Planning/Target Pointing/MATLAB Function ==
  data: Re input; r_target_ecef output; target_lat input; target_lon input
function r_target_ecef = fcn(Re, target_lat, target_lon)

lat = deg2rad(target_lat);
lon = deg2rad(target_lon);

x_ecef = Re * cos(lat) * cos(lon);
y_ecef = Re * cos(lat) * sin(lon);
z_ecef = Re * sin(lat);

r_target_ecef = [x_ecef; y_ecef; z_ecef];

== matlab function ADCS_onOrbit_TrueState/OBC/MATLAB Function ==
  data: internal input; mode output; fromTable input; wheelsEnable output; rodsEnable output
function [mode, wheelsEnable, rodsEnable] = fcn(internal, fromTable)

if internal ~= 2
    mode = internal;
    wheelsEnable    = 1;
    rodsEnable      = 1;
else
    mode            = fromTable(1);
    wheelsEnable    = fromTable(3);
    rodsEnable      = fromTable(2);
end

end
